simulink model "simscape_3link_flexjoint_sim"  (R2018b)
settings: Solver=ode45  StartTime=0.0  StopTime=T  FixedStep=0.1  MaxStep=0.05  RelTol=1e-3  EnableMultiTasking=on
values from neighbouring files (symbols this model uses):
  bl = [0.2;0.2;0.2]    [simscape_NE_comparison.m]    (also in simscape_NE_flexjoint_comparison.m; simscape_example.m; simscape_flexjoint_example.m)
  bm = [0.03;0.03;0.03]    [simscape_NE_flexjoint_comparison.m]    (also in simscape_flexjoint_example.m)
  csim = c    [simscape_NE_comparison.m]    (also in simscape_NE_flexjoint_comparison.m; simscape_example.m; simscape_flexjoint_example.m)
  d1 = 0.35    [simscape_NE_comparison.m]    (also in simscape_NE_flexjoint_comparison.m; simscape_example.m; simscape_flexjoint_example.m)
  d2 = 0.1    [simscape_NE_comparison.m]    (also in simscape_NE_flexjoint_comparison.m; simscape_example.m; simscape_flexjoint_example.m)
  d3 = 0.25    [simscape_NE_comparison.m]    (also in simscape_NE_flexjoint_comparison.m; simscape_example.m; simscape_flexjoint_example.m)
  Im = [0.4; 0.35; 0.28]    [simscape_NE_flexjoint_comparison.m]    (also in simscape_flexjoint_example.m)
  Isim = Ic    [simscape_NE_comparison.m]    (also in simscape_NE_flexjoint_comparison.m; simscape_example.m; simscape_flexjoint_example.m)
  K = [50; 20; 15]    [simscape_NE_flexjoint_comparison.m]    (also in simscape_flexjoint_example.m)
  m = [3; 1.1; 2.4]    [simscape_NE_comparison.m]    (also in simscape_NE_flexjoint_comparison.m; simscape_example.m; simscape_flexjoint_example.m)
  N = [5; 3.3; 2.1]    [simscape_NE_flexjoint_comparison.m]    (also in simscape_flexjoint_example.m)
  q0 = [0.3;-0.1;-.21]    [simscape_NE_comparison.m]    (also in simscape_NE_flexjoint_comparison.m = [0.5;-0.22;0.06]; simscape_example.m = [0;0;0]; simscape_flexjoint_example.m = [0;0;0])
  qdot0 = [0.03;0.004;-0.1]    [simscape_NE_comparison.m]    (also in simscape_NE_flexjoint_comparison.m = [0.01;0.02;-0.015]; simscape_example.m = [0;0;0]; simscape_flexjoint_example.m = [0;0;0])
  qm0 = N.*q0    [simscape_NE_flexjoint_comparison.m]    (also in simscape_flexjoint_example.m)
  qmdot0 = N.*qdot0    [simscape_NE_flexjoint_comparison.m]    (also in simscape_flexjoint_example.m)
  taustep = [3;-3;2]    [simscape_NE_comparison.m]    (also in simscape_NE_flexjoint_comparison.m = [1;-1.4;0.7]; simscape_example.m = [0;0;0]; simscape_flexjoint_example.m = [0;0;0])
undefined symbols (not defined in the file or in its folder): X, Y, Z
libraries: nesl_utility x13, sm_lib x13
settings Model: Creator=davidcarabis  LastModifiedBy=davidcarabis
settings DataIOCC: LimitDataPoints=on
settings OptimizationCC: LifeSpan=inf
settings DebuggingCC: AllowSymbolicDim=off  SFUnexpectedBacktrackingDiag=warning  SFNoUnconditionalDefaultTransitionDiag=warning  SFExecutionAtInitializationDiag=none
settings SFSimCC: SimUseLocalCustomCode=off
settings RTWCC: RTWUseLocalCustomCode=off
settings CodeAppCC: StateflowObjectComments=on
settings GRTTargetCC: TargetLangStandard=C89/C90 (ANSI)  GeneratePreprocessorConditionals=Disable all
settings ConfigComp: CovMetricSettings=dw  CovHtmlReporting=on  CovSaveCumulativeToWorkspaceVar=on  CovSaveSingleToWorkspaceVar=on  CovExternalEMLEnable=off  CovSFcnEnable=off
settings SimscapeCC: SimscapeNominalValues="[{\"value\":\"10\",\"unit\":\"V\"},{\"value\":\"1\",\"unit\":\"A\"},{\"value\":\"10\",\"unit\":\"N*m\"},{\"value\":\"10\",\"unit\":\"bar\"},{\"value\":\"100\",\"unit\":\"kJ/kg\"},{\"value\":\"1\",\"unit\":\"kW\"},{\"value\":\"300\",\"unit\":\"K\"},{\"value\":\"100\",\"unit\":\"cm^3/s\"},{\"value\":\"1\",\"unit\":\"kN\"},{\"value\":\"1\",\"unit\":\"g/cm^3\"},{\"value\":\"1\",\"unit\":\"l\"},{\"value\":\"1\",\"unit\":\"cm^2\"},{\"value\":\"60\",\"unit\":\"Hz\"}]"  SimscapeLogType=all  SimscapeLogDataHistory=10000
settings ConfigurationSet: Description=SimMechanics 2G

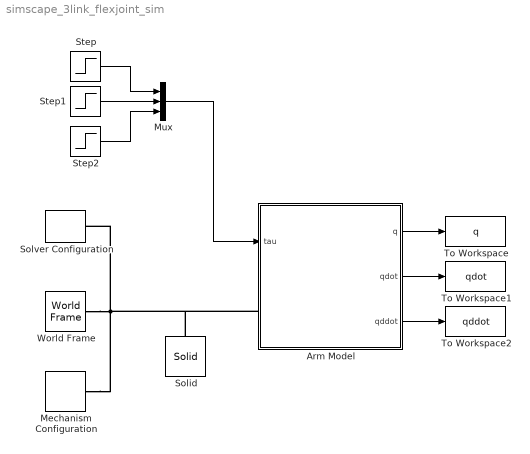
== system simscape_3link_flexjoint_sim ==
  Arm Model : Subsystem
  Mechanism Configuration : sm_lib/Utilities/Mechanism Configuration  UniformGravity=Constant  GravityVector=g  GravityUnits=m/s^2  LinearizationDelta=0.001
  Mux : Mux  Inputs=3
  Solid : sm_lib/Body Elements/Solid  InertiaType=CalculateFromGeometry  Mass=1  MassUnits=kg  CenterOfMass=[0 0 0]  CenterOfMassUnits=m  MomentsOfInertia=[1 1 1]  MomentsOfInertiaUnits=kg*m^2  ProductsOfInertia=[0 0 0]  ProductsOfInertiaUnits=kg*m^2  BasedOnType=Density  Density=1000  DensityUnits=kg/m^3  DoExposeReferenceFrame=on  SerializedFrames=<Frames/>  GraphicType=FromGeometry  MarkerShape=Sphere  MarkerSize=10  GraphicVisPropType=SimpleVisualProperties  GraphicDiffuseColor=[0.5 0.5 0.5]  GraphicSpecularColor=[0.5 0.5 0.5 1.0]  GraphicAmbientColor=[0.15 0.15 0.15 1.0]  GraphicEmissiveColor=[0.0 0.0 0.0 1.0]  GraphicShininess=75  GraphicOpacity=1.0  GeometryShape=Brick  RectangleSize=[1 1]  RectangleSizeUnits=m  BrickDimensions=[1 1 0.1]  BrickDimensionUnits=m  CylinderRadius=1  CylinderRadiusUnits=m  CylinderLength=1  CylinderLengthUnits=m  SphereRadius=1  SphereRadiusUnits=m  EllipsoidRadii=[1 1 1]  EllipsoidRadiiUnits=m  ExtrusionCrossSection=[1 1; -1 1; -1 -1; 1 -1]  ExtrusionCrossSectionUnits=m  ExtrusionLength=1  ExtrusionLengthUnits=m  PolygonNumSides=3  PolygonOuterRadius=1  PolygonOuterRadiusUnits=m  ExtGeomFileType=STEP  ExtGeomFileUnits=m  RevolutionCrossSection=[1 1; 1 -1; 2 -1; 2 1]  RevolutionCrossSectionUnits=m  RevolutionExtent=Full  RevolutionAngle=180  RevolutionAngleUnits=deg
  Solver Configuration : nesl_utility/Solver Configuration  PhysicalDomain=network_engine_domain  SubClassName=solver  LeftPortType=input  RightPortType=generic  Tones=[]  Harmonics=[]  SimulateNoise=off  Profile=off  UseLocalSampling=off  EnableSwitchedLinearOptims=on  FrequencyDomain=off  UseCCode=off  RelTol=0.001  AbsTol=1e-06  MinStep=1e-09  ToWorkspace=off  RevertToSquareIcSolve=off  NumHomotopyIterations=100  PhasorMode=off  PhasorModeNumHarmonics=1  DoDC=off  ResidualTolerance=1e-09  UseLocalSolver=off  LocalSolverChoice=NE_BACKWARD_EULER_ADVANCER  LocalSolverSampleTime=0.001  DoFixedCost=off  MaxNonlinIter=3  MaxModeIter=2  LinearAlgebra=Sparse  EquationFormulation=NE_TIME_EF  DelaysMemoryBudget=1024  AutomaticFiltering=on  FilteringTimeConstant=0.001  PartitionStorageMethod=AS_NEEDED  PartitionMemoryBudget=1024
  Step : Step  Time=0.5  Before=taustep(1)  After=0  SampleTime=0
  Step1 : Step  Time=0.5  Before=taustep(2)  After=0  SampleTime=0
  Step2 : Step  Time=0.5  Before=taustep(3)  After=0  SampleTime=0
  To Workspace : ToWorkspace  VariableName=q  SampleTime=-1
  To Workspace1 : ToWorkspace  VariableName=qdot  SampleTime=-1
  To Workspace2 : ToWorkspace  VariableName=qddot  SampleTime=-1
  World Frame : sm_lib/Frames and Transforms/World Frame
  wires:
  Arm Model/1(q) -> To Workspace/1
  Arm Model/3(qddot) -> To Workspace2/1
  Arm Model/2(qdot) -> To Workspace1/1
  Mux/1 -> Arm Model/1(tau)
  Step/1 -> Mux/1
  Step1/1 -> Mux/2
  Step2/1 -> Mux/3
  connections:
  Mechanism Configuration/RConn1 -- Solid/RConn1 -- Arm Model/LConn1 -- Solver Configuration/RConn1 -- World Frame/RConn1

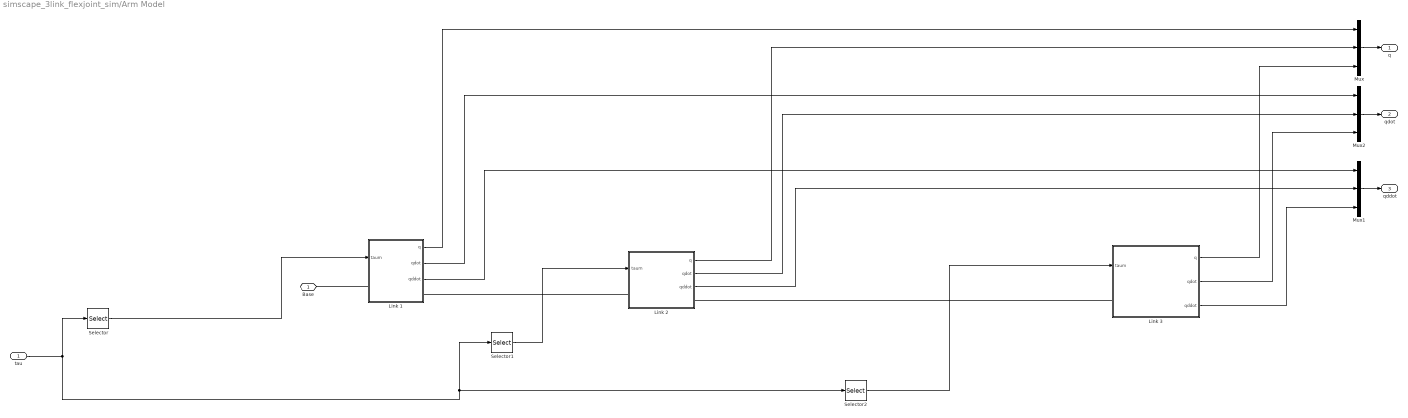
== system simscape_3link_flexjoint_sim/Arm Model ==
  tau : Inport
  Link 1 : Subsystem
  Link 2 : Subsystem
  Link 3 : Subsystem
  Mux : Mux  Inputs=3
  Mux1 : Mux  Inputs=3
  Mux2 : Mux  Inputs=3
  Selector : Selector  InputPortWidth=3  IndexOptions=Index vector (dialog)  Indices=[1]  OutputSizes=1
  Selector1 : Selector  InputPortWidth=3  IndexOptions=Index vector (dialog)  Indices=[2]  OutputSizes=1
  Selector2 : Selector  InputPortWidth=3  IndexOptions=Index vector (dialog)  Indices=[3]  OutputSizes=1
  Base : PMIOPort  Side=Left
  q : Outport
  qdot : Outport  Port=2
  qddot : Outport  Port=3
  wires:
  tau/1 -> Selector2/1, Selector1/1, Selector/1
  Link 1/3(qddot) -> Mux1/1
  Mux/1 -> q/1
  Mux2/1 -> qdot/1
  Mux1/1 -> qddot/1
  Selector/1 -> Link 1/1(taum)
  Link 1/1(q) -> Mux/1
  Link 1/2(qdot) -> Mux2/1
  Selector1/1 -> Link 2/1(taum)
  Link 2/1(q) -> Mux/2
  Link 2/2(qdot) -> Mux2/2
  Link 2/3(qddot) -> Mux1/2
  Selector2/1 -> Link 3/1(taum)
  Link 3/1(q) -> Mux/3
  Link 3/2(qdot) -> Mux2/3
  Link 3/3(qddot) -> Mux1/3
  connections:
  Link 1/LConn1 -- Base/RConn1
  Link 2/LConn1 -- Link 1/RConn1
  Link 3/LConn1 -- Link 2/RConn1

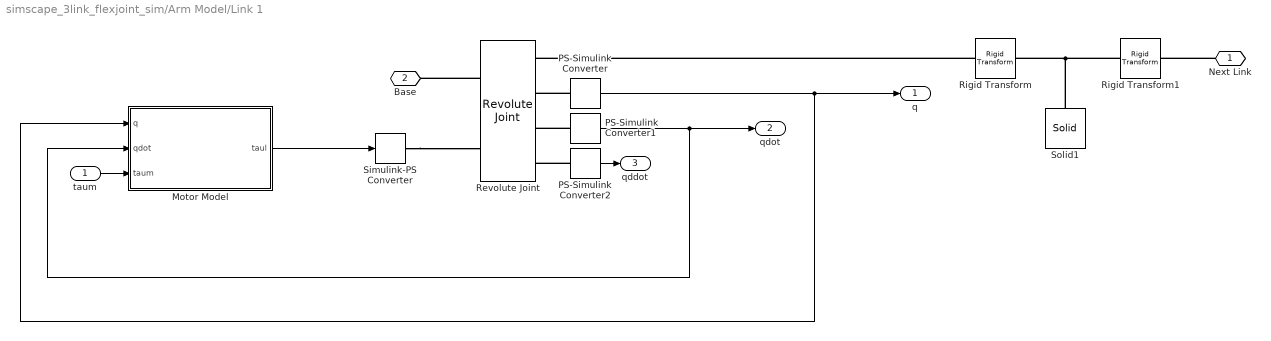
== system simscape_3link_flexjoint_sim/Arm Model/Link 1 ==
  taum : Inport
  Motor Model : Subsystem
  PS-Simulink Converter : nesl_utility/PS-Simulink Converter  PhysicalDomain=network_engine_domain  SubClassName=ps_output  LeftPortType=input  RightPortType=output  PseudoPeriodic=off  Frequencies=[]  Unit=1  AffineConversion=off
  PS-Simulink Converter1 : nesl_utility/PS-Simulink Converter  PhysicalDomain=network_engine_domain  SubClassName=ps_output  LeftPortType=input  RightPortType=output  PseudoPeriodic=off  Frequencies=[]  Unit=1  AffineConversion=off
  PS-Simulink Converter2 : nesl_utility/PS-Simulink Converter  PhysicalDomain=network_engine_domain  SubClassName=ps_output  LeftPortType=input  RightPortType=output  PseudoPeriodic=off  Frequencies=[]  Unit=1  AffineConversion=off
  Revolute Joint : sm_lib/Joints/Revolute Joint  SenseConstraintForce=off  SenseConstraintForceX=off  SenseConstraintForceY=off  SenseConstraintForceZ=off  SenseConstraintTorque=off  SenseConstraintTorqueX=off  SenseConstraintTorqueY=off  SenseConstraintTorqueZ=off  SenseTotalForce=off  SenseTotalForceX=off  SenseTotalForceY=off  SenseTotalForceZ=off  SenseTotalTorque=off  SenseTotalTorqueX=off  SenseTotalTorqueY=off  SenseTotalTorqueZ=off  CompositeWrenchDir=FollowerOnBase  CompositeWrenchFrame=BaseFrame  EquilibriumPosition=0  EquilibriumPositionUnits=deg  SpringStiffness=0  SpringStiffnessUnits=N*m/deg  DampingCoefficient=0  DampingCoefficientUnits=N*m/(rad/s)  TorqueActuationMode=InputTorque  MotionActuationMode=ComputedMotion  SensePosition=on  SenseVelocity=on  SenseAcceleration=on  SenseTorqueForce=off  PositionTargetSpecify=on  PositionTargetPriority=High  PositionTargetValue=q0(1)  PositionTargetValueUnits=rad  VelocityTargetSpecify=on  VelocityTargetPriority=High  VelocityTargetValue=qdot0(1)  VelocityTargetValueUnits=rad/s
  Rigid Transform : sm_lib/Frames and Transforms/Rigid Transform  TranslationMethod=Cartesian  TranslationStandardOffset=0  TranslationLengthUnit=m  TranslationStandardAxis=+Z  TranslationCartesianOffset=[0;0;d1/2]  TranslationROffset=0  TranslationROffsetUnits=m  TranslationZOffset=0  TranslationZOffsetUnits=m  TranslationThetaOffset=0  TranslationThetaOffsetUnits=deg  RotationMethod=None  RotationAngleUnits=deg  RotationStandardAxis=+Z  RotationAngle=0.0  RotationArbitraryAxis=[0 0 1]  FollAlignAxisA=+X  BaseAlignAxisA=+Y  FollAlignAxisB=+Y  BaseAlignAxisB=+Z  RotationSequenceAxes=FollowerAxes  RotationSequence=XYX  RotationSequenceAngles=[0 0 0]  RotationSequenceAnglesUnits=deg  RotationMatrix=[1 0 0; 0 1 0; 0 0 1]
  Rigid Transform1 : sm_lib/Frames and Transforms/Rigid Transform  TranslationMethod=Cartesian  TranslationStandardOffset=0  TranslationLengthUnit=m  TranslationStandardAxis=+Z  TranslationCartesianOffset=[0;0;d1/2]  TranslationROffset=0  TranslationROffsetUnits=m  TranslationZOffset=0  TranslationZOffsetUnits=m  TranslationThetaOffset=0  TranslationThetaOffsetUnits=deg  RotationMethod=StandardAxis  RotationAngleUnits=rad  RotationStandardAxis=-X  RotationAngle=pi/2  RotationArbitraryAxis=[0 0 1]  FollAlignAxisA=+X  BaseAlignAxisA=+Y  FollAlignAxisB=+Y  BaseAlignAxisB=+Z  RotationSequenceAxes=FollowerAxes  RotationSequence=XYX  RotationSequenceAngles=[0 0 0]  RotationSequenceAnglesUnits=deg  RotationMatrix=[1 0 0; 0 1 0; 0 0 1]
  Simulink-PS Converter : nesl_utility/Simulink-PS Converter  PhysicalDomain=network_engine_domain  SubClassName=ps_input  LeftPortType=input  RightPortType=output  PseudoPeriodic=off  Frequencies=[]  NoiseDistribution=none  NoiseParameters=[]  Unit=1  AffineConversion=off  FilteringAndDerivatives=zero  SimscapeFilterOrder=1  InputFilterTimeConstant=0.001  UdotUserProvided=1
  Solid1 : sm_lib/Body Elements/Solid  InertiaType=Custom  Mass=m(1)  MassUnits=kg  CenterOfMass=-[0;0;d1/2] + csim(:,1)  CenterOfMassUnits=m  MomentsOfInertia=[Isim(1,1,1), Isim(2,2,1), Isim(3,3,1)]  MomentsOfInertiaUnits=kg*m^2  ProductsOfInertia=[Isim(2,3,1), Isim(3,1,1), Isim(1,2,1)]  ProductsOfInertiaUnits=kg*m^2  BasedOnType=Density  Density=1000  DensityUnits=kg/m^3  DoExposeReferenceFrame=on  SerializedFrames=<Frames/>  GraphicType=FromGeometry  MarkerShape=Sphere  MarkerSize=10  GraphicVisPropType=SimpleVisualProperties  GraphicDiffuseColor=[0.2 0.2 1.0]  GraphicSpecularColor=[0.5 0.5 0.5 1.0]  GraphicAmbientColor=[0.15 0.15 0.15 1.0]  GraphicEmissiveColor=[0.0 0.0 0.0 1.0]  GraphicShininess=75  GraphicOpacity=1.0  GeometryShape=Cylinder  RectangleSize=[1 1]  RectangleSizeUnits=m  BrickDimensions=[1 1 0.1]  BrickDimensionUnits=m  CylinderRadius=r  CylinderRadiusUnits=m  CylinderLength=d1  CylinderLengthUnits=m  SphereRadius=1  SphereRadiusUnits=m  EllipsoidRadii=[1 1 1]  EllipsoidRadiiUnits=m  ExtrusionCrossSection=[1 1; -1 1; -1 -1; 1 -1]  ExtrusionCrossSectionUnits=m  ExtrusionLength=1  ExtrusionLengthUnits=m  PolygonNumSides=3  PolygonOuterRadius=1  PolygonOuterRadiusUnits=m  ExtGeomFileType=STEP  ExtGeomFileUnits=m  RevolutionCrossSection=[1 1; 1 -1; 2 -1; 2 1]  RevolutionCrossSectionUnits=m  RevolutionExtent=Full  RevolutionAngle=180  RevolutionAngleUnits=deg
  Next Link : PMIOPort  Side=Right
  Base : PMIOPort  Port=2  Side=Left
  q : Outport
  qdot : Outport  Port=2
  qddot : Outport  Port=3
  wires:
  PS-Simulink Converter/1 -> q/1, Motor Model/1(q)
  PS-Simulink Converter1/1 -> Motor Model/2(qdot), qdot/1
  Motor Model/1(taul) -> Simulink-PS Converter/1
  taum/1 -> Motor Model/3(taum)
  PS-Simulink Converter2/1 -> qddot/1
  connections:
  Next Link/RConn1 -- Rigid Transform1/RConn1
  Solid1/RConn1 -- Rigid Transform1/LConn1 -- Rigid Transform/RConn1
  Rigid Transform/LConn1 -- Revolute Joint/RConn1
  Simulink-PS Converter/RConn1 -- Revolute Joint/LConn2
  PS-Simulink Converter1/LConn1 -- Revolute Joint/RConn3
  PS-Simulink Converter/LConn1 -- Revolute Joint/RConn2
  Revolute Joint/LConn1 -- Base/RConn1
  PS-Simulink Converter2/LConn1 -- Revolute Joint/RConn4

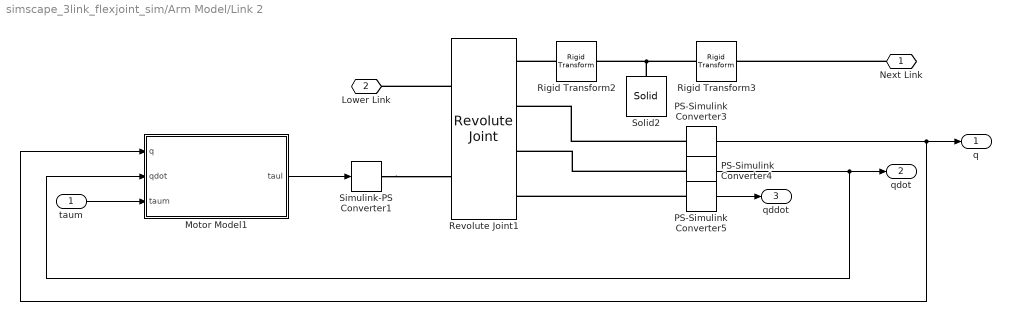
== system simscape_3link_flexjoint_sim/Arm Model/Link 2 ==
  taum : Inport
  Motor Model1 : Subsystem
  PS-Simulink Converter3 : nesl_utility/PS-Simulink Converter  PhysicalDomain=network_engine_domain  SubClassName=ps_output  LeftPortType=input  RightPortType=output  PseudoPeriodic=off  Frequencies=[]  Unit=1  AffineConversion=off
  PS-Simulink Converter4 : nesl_utility/PS-Simulink Converter  PhysicalDomain=network_engine_domain  SubClassName=ps_output  LeftPortType=input  RightPortType=output  PseudoPeriodic=off  Frequencies=[]  Unit=1  AffineConversion=off
  PS-Simulink Converter5 : nesl_utility/PS-Simulink Converter  PhysicalDomain=network_engine_domain  SubClassName=ps_output  LeftPortType=input  RightPortType=output  PseudoPeriodic=off  Frequencies=[]  Unit=1  AffineConversion=off
  Revolute Joint1 : sm_lib/Joints/Revolute Joint  SenseConstraintForce=off  SenseConstraintForceX=off  SenseConstraintForceY=off  SenseConstraintForceZ=off  SenseConstraintTorque=off  SenseConstraintTorqueX=off  SenseConstraintTorqueY=off  SenseConstraintTorqueZ=off  SenseTotalForce=off  SenseTotalForceX=off  SenseTotalForceY=off  SenseTotalForceZ=off  SenseTotalTorque=off  SenseTotalTorqueX=off  SenseTotalTorqueY=off  SenseTotalTorqueZ=off  CompositeWrenchDir=FollowerOnBase  CompositeWrenchFrame=BaseFrame  EquilibriumPosition=0  EquilibriumPositionUnits=deg  SpringStiffness=0  SpringStiffnessUnits=N*m/deg  DampingCoefficient=0  DampingCoefficientUnits=N*m/(rad/s)  TorqueActuationMode=InputTorque  MotionActuationMode=ComputedMotion  SensePosition=on  SenseVelocity=on  SenseAcceleration=on  SenseTorqueForce=off  PositionTargetSpecify=on  PositionTargetPriority=High  PositionTargetValue=q0(2)  PositionTargetValueUnits=rad  VelocityTargetSpecify=on  VelocityTargetPriority=High  VelocityTargetValue=qdot0(2)  VelocityTargetValueUnits=rad/s
  Rigid Transform2 : sm_lib/Frames and Transforms/Rigid Transform  TranslationMethod=Cartesian  TranslationStandardOffset=0  TranslationLengthUnit=m  TranslationStandardAxis=+Z  TranslationCartesianOffset=[0;0;d2/2]  TranslationROffset=0  TranslationROffsetUnits=m  TranslationZOffset=0  TranslationZOffsetUnits=m  TranslationThetaOffset=0  TranslationThetaOffsetUnits=deg  RotationMethod=None  RotationAngleUnits=rad  RotationStandardAxis=-X  RotationAngle=pi/2  RotationArbitraryAxis=[0 0 1]  FollAlignAxisA=+X  BaseAlignAxisA=+Y  FollAlignAxisB=+Y  BaseAlignAxisB=+Z  RotationSequenceAxes=FollowerAxes  RotationSequence=XYX  RotationSequenceAngles=[0 0 0]  RotationSequenceAnglesUnits=deg  RotationMatrix=[1 0 0; 0 1 0; 0 0 1]
  Rigid Transform3 : sm_lib/Frames and Transforms/Rigid Transform  TranslationMethod=Cartesian  TranslationStandardOffset=0  TranslationLengthUnit=m  TranslationStandardAxis=+Z  TranslationCartesianOffset=[0;-d3/2;d2/2]  TranslationROffset=0  TranslationROffsetUnits=m  TranslationZOffset=0  TranslationZOffsetUnits=m  TranslationThetaOffset=0  TranslationThetaOffsetUnits=deg  RotationMethod=StandardAxis  RotationAngleUnits=rad  RotationStandardAxis=+X  RotationAngle=pi/2  RotationArbitraryAxis=[0 0 1]  FollAlignAxisA=+X  BaseAlignAxisA=+Y  FollAlignAxisB=+Y  BaseAlignAxisB=+Z  RotationSequenceAxes=FollowerAxes  RotationSequence=XYX  RotationSequenceAngles=[0 0 0]  RotationSequenceAnglesUnits=deg  RotationMatrix=[1 0 0; 0 1 0; 0 0 1]
  Simulink-PS Converter1 : nesl_utility/Simulink-PS Converter  PhysicalDomain=network_engine_domain  SubClassName=ps_input  LeftPortType=input  RightPortType=output  PseudoPeriodic=off  Frequencies=[]  NoiseDistribution=none  NoiseParameters=[]  Unit=1  AffineConversion=off  FilteringAndDerivatives=zero  SimscapeFilterOrder=1  InputFilterTimeConstant=0.001  UdotUserProvided=1
  Solid2 : sm_lib/Body Elements/Solid  InertiaType=Custom  Mass=m(2)  MassUnits=kg  CenterOfMass=-[0;0;d2/2] + csim(:,2)  CenterOfMassUnits=m  MomentsOfInertia=[Isim(1,1,2), Isim(2,2,2), Isim(3,3,2)]  MomentsOfInertiaUnits=kg*m^2  ProductsOfInertia=[Isim(2,3,2), Isim(3,1,2), Isim(1,2,2)]  ProductsOfInertiaUnits=kg*m^2  BasedOnType=Density  Density=1000  DensityUnits=kg/m^3  DoExposeReferenceFrame=on  SerializedFrames=<Frames/>  GraphicType=FromGeometry  MarkerShape=Sphere  MarkerSize=10  GraphicVisPropType=SimpleVisualProperties  GraphicDiffuseColor=[0.2 0.2 1.0]  GraphicSpecularColor=[0.5 0.5 0.5 1.0]  GraphicAmbientColor=[0.15 0.15 0.15 1.0]  GraphicEmissiveColor=[0.0 0.0 0.0 1.0]  GraphicShininess=75  GraphicOpacity=1.0  GeometryShape=Cylinder  RectangleSize=[1 1]  RectangleSizeUnits=m  BrickDimensions=[1 1 0.1]  BrickDimensionUnits=m  CylinderRadius=r  CylinderRadiusUnits=m  CylinderLength=d2  CylinderLengthUnits=m  SphereRadius=1  SphereRadiusUnits=m  EllipsoidRadii=[1 1 1]  EllipsoidRadiiUnits=m  ExtrusionCrossSection=[1 1; -1 1; -1 -1; 1 -1]  ExtrusionCrossSectionUnits=m  ExtrusionLength=1  ExtrusionLengthUnits=m  PolygonNumSides=3  PolygonOuterRadius=1  PolygonOuterRadiusUnits=m  ExtGeomFileType=STEP  ExtGeomFileUnits=m  RevolutionCrossSection=[1 1; 1 -1; 2 -1; 2 1]  RevolutionCrossSectionUnits=m  RevolutionExtent=Full  RevolutionAngle=180  RevolutionAngleUnits=deg
  Next Link : PMIOPort  Side=Right
  Lower Link : PMIOPort  Port=2  Side=Left
  q : Outport
  qdot : Outport  Port=2
  qddot : Outport  Port=3
  wires:
  PS-Simulink Converter5/1 -> qddot/1
  Motor Model1/1(taul) -> Simulink-PS Converter1/1
  taum/1 -> Motor Model1/3(taum)
  PS-Simulink Converter4/1 -> qdot/1, Motor Model1/2(qdot)
  PS-Simulink Converter3/1 -> Motor Model1/1(q), q/1
  connections:
  Revolute Joint1/LConn1 -- Lower Link/RConn1
  PS-Simulink Converter5/LConn1 -- Revolute Joint1/RConn4
  Simulink-PS Converter1/RConn1 -- Revolute Joint1/LConn2
  Solid2/RConn1 -- Rigid Transform3/LConn1 -- Rigid Transform2/RConn1
  PS-Simulink Converter3/LConn1 -- Revolute Joint1/RConn2
  Next Link/RConn1 -- Rigid Transform3/RConn1
  PS-Simulink Converter4/LConn1 -- Revolute Joint1/RConn3
  Rigid Transform2/LConn1 -- Revolute Joint1/RConn1

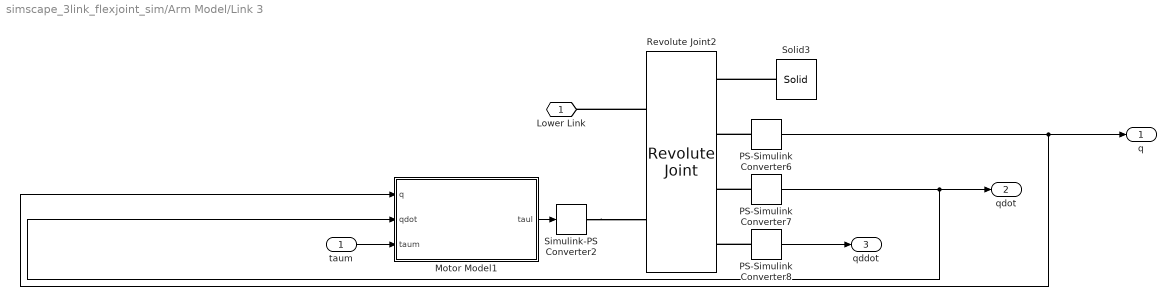
== system simscape_3link_flexjoint_sim/Arm Model/Link 3 ==
  taum : Inport
  Motor Model1 : Subsystem
  PS-Simulink Converter6 : nesl_utility/PS-Simulink Converter  PhysicalDomain=network_engine_domain  SubClassName=ps_output  LeftPortType=input  RightPortType=output  PseudoPeriodic=off  Frequencies=[]  Unit=1  AffineConversion=off
  PS-Simulink Converter7 : nesl_utility/PS-Simulink Converter  PhysicalDomain=network_engine_domain  SubClassName=ps_output  LeftPortType=input  RightPortType=output  PseudoPeriodic=off  Frequencies=[]  Unit=1  AffineConversion=off
  PS-Simulink Converter8 : nesl_utility/PS-Simulink Converter  PhysicalDomain=network_engine_domain  SubClassName=ps_output  LeftPortType=input  RightPortType=output  PseudoPeriodic=off  Frequencies=[]  Unit=1  AffineConversion=off
  Revolute Joint2 : sm_lib/Joints/Revolute Joint  SenseConstraintForce=off  SenseConstraintForceX=off  SenseConstraintForceY=off  SenseConstraintForceZ=off  SenseConstraintTorque=off  SenseConstraintTorqueX=off  SenseConstraintTorqueY=off  SenseConstraintTorqueZ=off  SenseTotalForce=off  SenseTotalForceX=off  SenseTotalForceY=off  SenseTotalForceZ=off  SenseTotalTorque=off  SenseTotalTorqueX=off  SenseTotalTorqueY=off  SenseTotalTorqueZ=off  CompositeWrenchDir=FollowerOnBase  CompositeWrenchFrame=BaseFrame  EquilibriumPosition=0  EquilibriumPositionUnits=deg  SpringStiffness=0  SpringStiffnessUnits=N*m/deg  DampingCoefficient=0  DampingCoefficientUnits=N*m/(rad/s)  TorqueActuationMode=InputTorque  MotionActuationMode=ComputedMotion  SensePosition=on  SenseVelocity=on  SenseAcceleration=on  SenseTorqueForce=off  PositionTargetSpecify=on  PositionTargetPriority=High  PositionTargetValue=q0(3)  PositionTargetValueUnits=rad  VelocityTargetSpecify=on  VelocityTargetPriority=High  VelocityTargetValue=qdot0(3)  VelocityTargetValueUnits=rad/s
  Simulink-PS Converter2 : nesl_utility/Simulink-PS Converter  PhysicalDomain=network_engine_domain  SubClassName=ps_input  LeftPortType=input  RightPortType=output  PseudoPeriodic=off  Frequencies=[]  NoiseDistribution=none  NoiseParameters=[]  Unit=1  AffineConversion=off  FilteringAndDerivatives=zero  SimscapeFilterOrder=1  InputFilterTimeConstant=0.001  UdotUserProvided=1
  Solid3 : sm_lib/Body Elements/Solid  InertiaType=Custom  Mass=m(3)  MassUnits=kg  CenterOfMass=-[0;0;d3/2] + csim(:,3)  CenterOfMassUnits=m  MomentsOfInertia=[Isim(1,1,3), Isim(2,2,3), Isim(3,3,3)]  MomentsOfInertiaUnits=kg*m^2  ProductsOfInertia=[Isim(2,3,3), Isim(3,1,3), Isim(1,2,3)]  ProductsOfInertiaUnits=kg*m^2  BasedOnType=Density  Density=1000  DensityUnits=kg/m^3  DoExposeReferenceFrame=on  SerializedFrames=<Frames/>  GraphicType=FromGeometry  MarkerShape=Sphere  MarkerSize=10  GraphicVisPropType=SimpleVisualProperties  GraphicDiffuseColor=[0.2 0.2 1.0]  GraphicSpecularColor=[0.5 0.5 0.5 1.0]  GraphicAmbientColor=[0.15 0.15 0.15 1.0]  GraphicEmissiveColor=[0.0 0.0 0.0 1.0]  GraphicShininess=75  GraphicOpacity=1.0  GeometryShape=Cylinder  RectangleSize=[1 1]  RectangleSizeUnits=m  BrickDimensions=[1 1 0.1]  BrickDimensionUnits=m  CylinderRadius=r  CylinderRadiusUnits=m  CylinderLength=d3  CylinderLengthUnits=m  SphereRadius=1  SphereRadiusUnits=m  EllipsoidRadii=[1 1 1]  EllipsoidRadiiUnits=m  ExtrusionCrossSection=[1 1; -1 1; -1 -1; 1 -1]  ExtrusionCrossSectionUnits=m  ExtrusionLength=1  ExtrusionLengthUnits=m  PolygonNumSides=3  PolygonOuterRadius=1  PolygonOuterRadiusUnits=m  ExtGeomFileType=STEP  ExtGeomFileUnits=m  RevolutionCrossSection=[1 1; 1 -1; 2 -1; 2 1]  RevolutionCrossSectionUnits=m  RevolutionExtent=Full  RevolutionAngle=180  RevolutionAngleUnits=deg
  Lower Link : PMIOPort  Side=Left
  q : Outport
  qdot : Outport  Port=2
  qddot : Outport  Port=3
  wires:
  taum/1 -> Motor Model1/3(taum)
  PS-Simulink Converter7/1 -> qdot/1, Motor Model1/2(qdot)
  Motor Model1/1(taul) -> Simulink-PS Converter2/1
  PS-Simulink Converter6/1 -> q/1, Motor Model1/1(q)
  PS-Simulink Converter8/1 -> qddot/1
  connections:
  Revolute Joint2/LConn1 -- Lower Link/RConn1
  PS-Simulink Converter7/LConn1 -- Revolute Joint2/RConn3
  PS-Simulink Converter6/LConn1 -- Revolute Joint2/RConn2
  Solid3/RConn1 -- Revolute Joint2/RConn1
  Simulink-PS Converter2/RConn1 -- Revolute Joint2/LConn2
  PS-Simulink Converter8/LConn1 -- Revolute Joint2/RConn4

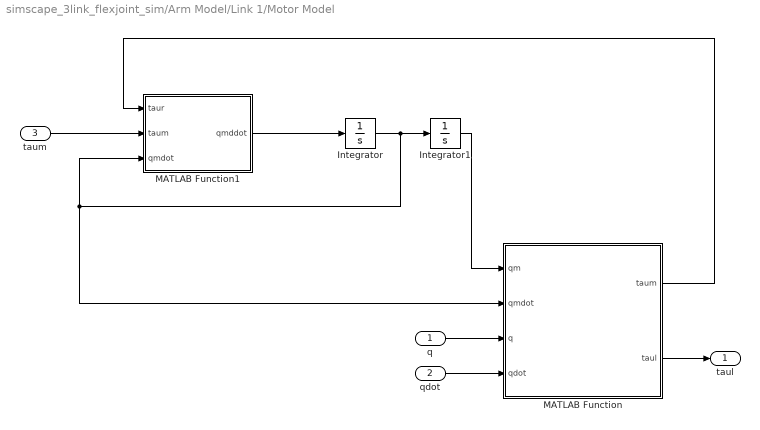
== system simscape_3link_flexjoint_sim/Arm Model/Link 1/Motor Model ==
  q : Inport
  qdot : Inport  Port=2
  taum : Inport  Port=3
  Integrator : Integrator  InitialCondition=qmdot0(1)
  Integrator1 : Integrator  InitialCondition=qm0(1)
  MATLAB Function : MATLAB Function  TreatAsAtomicUnit=on  mask{K=K(1), N=N(1), bl=bl(1), bm=bm(1)}
      mask prompts: K "Spring Constants"; N "Gear Ratio"; bl "Gear Damping"; bm "Motor Damping"
  MATLAB Function1 : MATLAB Function  TreatAsAtomicUnit=on  mask{bm=bm(1), Im=Im(1)}
      mask prompts: bm "Motor Friction"; Im "Motor Inertia"
  taul : Outport
  wires:
  q/1 -> MATLAB Function/3(q)
  qdot/1 -> MATLAB Function/4(qdot)
  MATLAB Function/2(taul) -> taul/1
  MATLAB Function/1(taum) -> MATLAB Function1/1(taur)
  MATLAB Function1/1(qmddot) -> Integrator/1
  Integrator1/1 -> MATLAB Function/1(qm)
  taum/1 -> MATLAB Function1/2(taum)
  Integrator/1 -> Integrator1/1, MATLAB Function/2(qmdot), MATLAB Function1/3(qmdot)

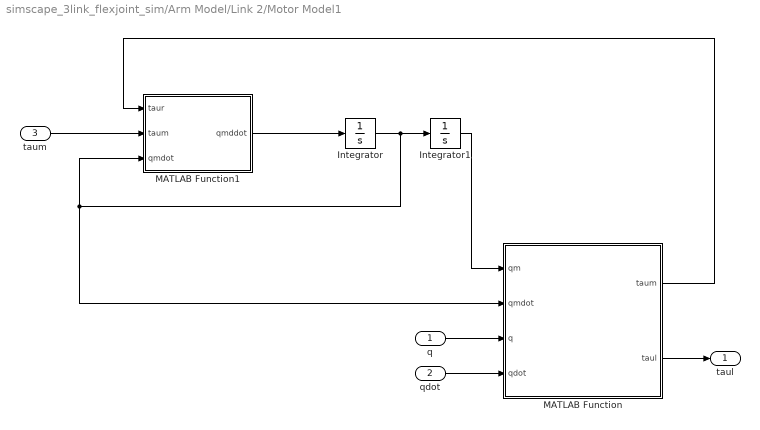
== system simscape_3link_flexjoint_sim/Arm Model/Link 2/Motor Model1 ==
  q : Inport
  qdot : Inport  Port=2
  taum : Inport  Port=3
  Integrator : Integrator  InitialCondition=qmdot0(2)
  Integrator1 : Integrator  InitialCondition=qm0(2)
  MATLAB Function : MATLAB Function  TreatAsAtomicUnit=on  mask{K=K(2), N=N(2), bl=bl(2), bm=bm(2)}
      mask prompts: K "Spring Constants"; N "Gear Ratio"; bl "Gear Damping"; bm "Motor Damping"
  MATLAB Function1 : MATLAB Function  TreatAsAtomicUnit=on  mask{bm=bm(2), Im=Im(2)}
      mask prompts: bm "Motor Friction"; Im "Motor Inertia"
  taul : Outport
  wires:
  q/1 -> MATLAB Function/3(q)
  qdot/1 -> MATLAB Function/4(qdot)
  MATLAB Function/2(taul) -> taul/1
  MATLAB Function/1(taum) -> MATLAB Function1/1(taur)
  MATLAB Function1/1(qmddot) -> Integrator/1
  Integrator1/1 -> MATLAB Function/1(qm)
  taum/1 -> MATLAB Function1/2(taum)
  Integrator/1 -> Integrator1/1, MATLAB Function/2(qmdot), MATLAB Function1/3(qmdot)

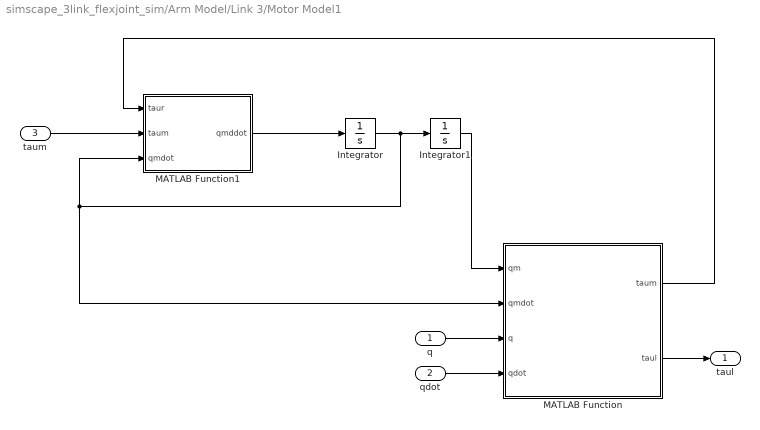
== system simscape_3link_flexjoint_sim/Arm Model/Link 3/Motor Model1 ==
  q : Inport
  qdot : Inport  Port=2
  taum : Inport  Port=3
  Integrator : Integrator  InitialCondition=qmdot0(3)
  Integrator1 : Integrator  InitialCondition=qm0(3)
  MATLAB Function : MATLAB Function  TreatAsAtomicUnit=on  mask{K=K(3), N=N(3), bl=bl(3), bm=bm(3)}
      mask prompts: K "Spring Constants"; N "Gear Ratio"; bl "Gear Damping"; bm "Motor Damping"
  MATLAB Function1 : MATLAB Function  TreatAsAtomicUnit=on  mask{bm=bm(3), Im=Im(3)}
      mask prompts: bm "Motor Friction"; Im "Motor Inertia"
  taul : Outport
  wires:
  q/1 -> MATLAB Function/3(q)
  qdot/1 -> MATLAB Function/4(qdot)
  MATLAB Function/2(taul) -> taul/1
  MATLAB Function/1(taum) -> MATLAB Function1/1(taur)
  MATLAB Function1/1(qmddot) -> Integrator/1
  Integrator1/1 -> MATLAB Function/1(qm)
  taum/1 -> MATLAB Function1/2(taum)
  Integrator/1 -> Integrator1/1, MATLAB Function/2(qmdot), MATLAB Function1/3(qmdot)

== matlab function simscape_3link_flexjoint_sim/Arm Model/Link 1/Motor Model/MATLAB Function1 ==
  data: taur input; taum input; qmddot output; qmdot input; bm parameter; Im parameter
function qmddot = fcn(taur, taum, qmdot, bm, Im)

qmddot =(taum + taur -bm*qmdot)/Im;

== matlab function simscape_3link_flexjoint_sim/Arm Model/Link 1/Motor Model/MATLAB Function ==
  data: qm input; taum output; qmdot input; q input; qdot input; taul output; K parameter; N parameter; bl parameter
function [taum,taul] = fcn(qm,qmdot,q,qdot,K, N, bl)

taum =  K./N.*(q - 1./N.*qm) + bl./N.*(qdot- 1./N.*qmdot);

taul = K.*(1./N.*qm - q) + bl.*(1./N.*qmdot - qdot);

== matlab function simscape_3link_flexjoint_sim/Arm Model/Link 2/Motor Model1/MATLAB Function ==
  data: qm input; taum output; qmdot input; q input; qdot input; taul output; K parameter; N parameter; bl parameter
function [taum,taul] = fcn(qm,qmdot,q,qdot,K, N, bl)

taum = K./N.*(q - 1./N.*qm) + bl./N.*(qdot- 1./N.*qmdot);

taul = K.*(1./N.*qm - q) + bl.*(1./N.*qmdot - qdot);

== matlab function simscape_3link_flexjoint_sim/Arm Model/Link 2/Motor Model1/MATLAB Function1 ==
  data: taur input; taum input; qmddot output; qmdot input; bm parameter; Im parameter
function qmddot = fcn(taur, taum, qmdot, bm, Im)

qmddot =(taum + taur -bm*qmdot)/Im;

== matlab function simscape_3link_flexjoint_sim/Arm Model/Link 3/Motor Model1/MATLAB Function ==
  data: qm input; taum output; qmdot input; q input; qdot input; taul output; K parameter; N parameter; bl parameter
function [taum,taul] = fcn(qm,qmdot,q,qdot,K, N, bl)

taum = K./N.*(q - 1./N.*qm) + bl./N.*(qdot- 1./N.*qmdot);

taul = K.*(1./N.*qm - q) + bl.*(1./N.*qmdot - qdot);

== matlab function simscape_3link_flexjoint_sim/Arm Model/Link 3/Motor Model1/MATLAB Function1 ==
  data: taur input; taum input; qmddot output; qmdot input; bm parameter; Im parameter
function qmddot = fcn(taur, taum, qmdot, bm, Im)

qmddot =(taum + taur -bm*qmdot)/Im;
